simulink model "Nomto Model"  (R2022a)
settings: Solver=VariableStepAuto  StartTime=0.0  StopTime=200  RelTol=1e-3
settings Model: Creator=Z0150218  LastModifiedBy=Z0150218

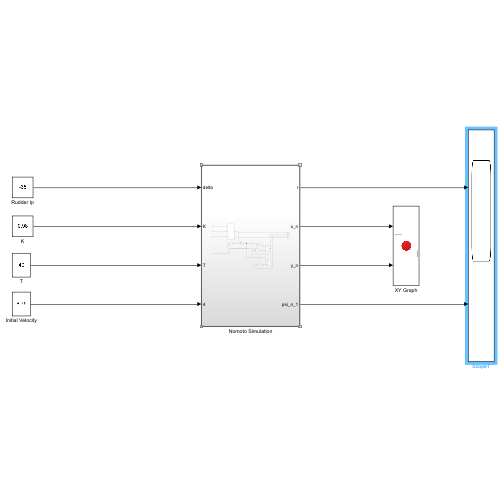
[thumbnail: Simulink's stored preview of the top-level diagram]
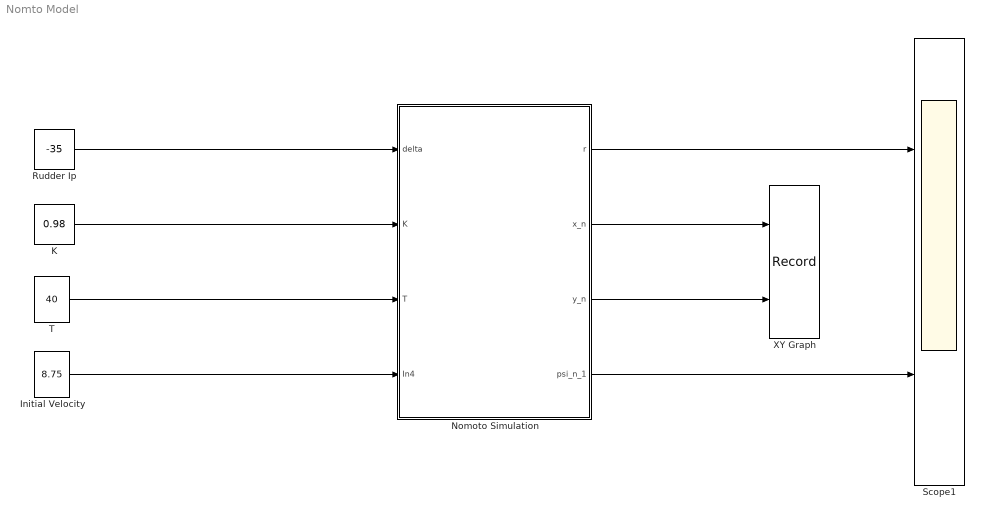
== system Nomto Model ==
  Initial Velocity : Constant  Value=8.75
  K : Constant  Value=0.98
  Nomoto Simulation : Subsystem
  Rudder Ip : Constant  Value=-35
  Scope1 : Scope  NumInputPorts=2
  T : Constant  Value=40
  XY Graph : Record  VariableName=X_Y_Position  RecordToWorkspace=on  FileSettingsInternal="{\"entries\":[{\"content\":{\"excelSettings\":{\"content\":{},\"type\":\"Streamout.ExcelSettings\"}},\"type\":\"Streamout.FileSettingStorage\",\"uuid\":\"6635f460-40b1-429d-8992-c5b395233bd7\"}],\"packageUris\":[\"http://schema.mathworks.com/mf0/streamout_blocks/R2020a\"],\"version\":\"1.0\"}"  Layout=[1 1]  SignalsInternal="{\"entries\":[{\"content\":{\"signals\":[{\"content\":{\"blockPath\":[\"model/XY Graph\"],\"channel\":[],\"dimensions\":[1],\"domain\":\"model/XY Graph\",\"lineColor\":\"#a2142f\",\"plots\":[1],\"port\":1,\"sid\":[\"\"],\"signalID\":43,\"signalName\":\"Nomoto Simulation:2\"},\"type\":\"RecordBlkView.Signal\",\"uuid\":\"2db5812d-c037-4b14-baed-b0e3edf6e0ba\"},{\"content\":{\"blockPath\":[\"model/XY Graph\"],\"channel\":[],\"dimensions\":[1],\"domain\":\"model/XY Graph\",\"lineColor\":\"#139fff\",\"plots\":[1],\"port\":2,\"sid\":[\"\"],\"signalID\":47,\"signalName\":\"Nomoto Simulation:3\"},\"type\":\"RecordBlkView.Signal\",\"uuid\":\"7fc5cd1a-1a78-4c0c-9b5d-9f5c7e47b2eb\"}]},\"type\":\"RecordBlkView.InputSignals\",\"uuid\":\"ea99f773-b7af-4dc6-9da2-234de1809b82\"}],\"packageUris\":[\"http://schema.mathworks.com/mf0/streamout_blocks/R2020a\"],\"version\":\"1.0\"}"  VisualizationBindings="{\"xyplotplugin\":{\"info\":[{\"series\":[{\"bindingParametersList\":[{\"parameter\":\"X-Axis\",\"signalID\":43,\"signalName\":\"Nomoto Simulation:2\"},{\"parameter\":\"Y-Axis\",\"signalID\":47,\"signalName\":\"Nomoto Simulation:3\"}],\"seriesID\":59298}],\"subplotID\":1}]}}"  CompatibilityTag=XY
  wires:
  Rudder Ip/1 -> Nomoto Simulation/1(delta)
  K/1 -> Nomoto Simulation/2(K)
  T/1 -> Nomoto Simulation/3(T)
  Initial Velocity/1 -> Nomoto Simulation/4(In4)
  Nomoto Simulation/4(psi_n_1) -> Scope1/2
  Nomoto Simulation/1(r) -> Scope1/1
  Nomoto Simulation/2(x_n) -> XY Graph/1
  Nomoto Simulation/3(y_n) -> XY Graph/2

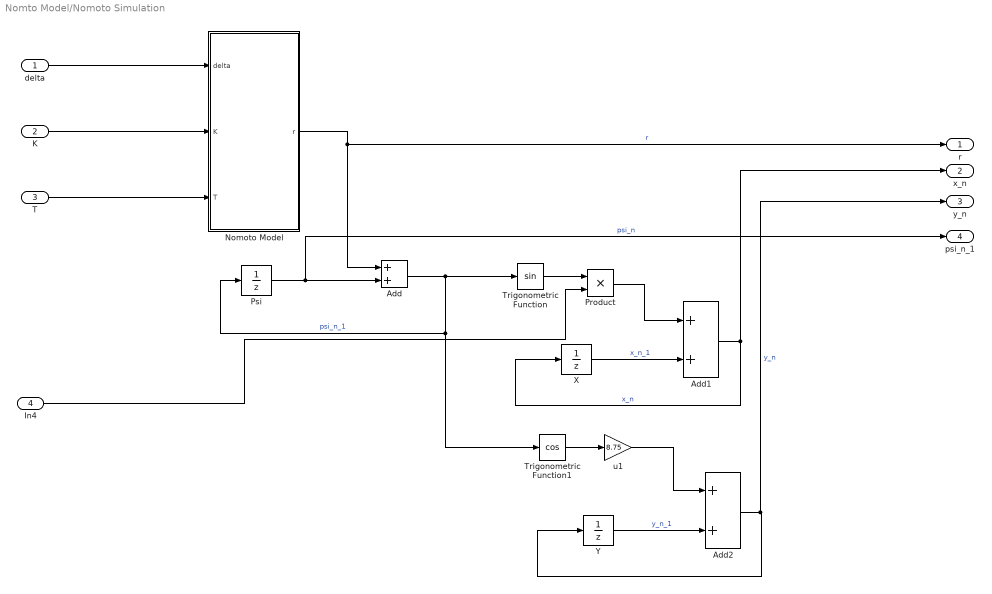
== system Nomto Model/Nomoto Simulation ==
  delta : Inport
  K : Inport  Port=2
  T : Inport  Port=3
  In4 : Inport  Port=4
  Add : Sum
  Add1 : Sum
  Add2 : Sum
  Nomoto Model : Subsystem
  Product : Product
  Psi : UnitDelay  SampleTime=-1  HasFrameUpgradeWarning=on
  Trigonometric Function : Trigonometry
  Trigonometric Function1 : Trigonometry  Operator=cos
  X : UnitDelay  SampleTime=-1  HasFrameUpgradeWarning=on
  Y : UnitDelay  SampleTime=-1  HasFrameUpgradeWarning=on
  u1 : Gain  Gain=8.75
  r : Outport
  x_n : Outport  Port=2
  y_n : Outport  Port=3
  psi_n_1 : Outport  Port=4
  wires:
  K/1 -> Nomoto Model/2(K)
  Add1/1 -> x_n/1, X/1  "x_n"
  Add/1 -> Trigonometric Function1/1, Psi/1, Trigonometric Function/1  "psi_n_1"
  Psi/1 -> psi_n_1/1, Add/2  "psi_n"
  Add2/1 -> y_n/1, Y/1  "y_n"
  Product/1 -> Add1/1
  Nomoto Model/1(r) -> r/1, Add/1  "r"
  In4/1 -> Product/2
  X/1 -> Add1/2  "x_n_1"
  Trigonometric Function/1 -> Product/1
  Trigonometric Function1/1 -> u1/1
  Y/1 -> Add2/2  "y_n_1"
  u1/1 -> Add2/1
  delta/1 -> Nomoto Model/1(delta)
  T/1 -> Nomoto Model/3(T)

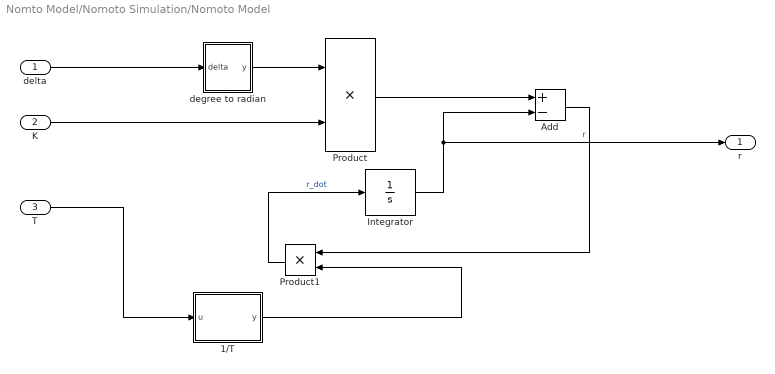
== system Nomto Model/Nomoto Simulation/Nomoto Model ==
  delta : Inport
  K : Inport  Port=2
  T : Inport  Port=3
  1/T : MATLAB Function  TreatAsAtomicUnit=on
  Add : Sum  Inputs=+-
  Integrator : Integrator
  Product : Product
  Product1 : Product
  degree to radian : MATLAB Function  TreatAsAtomicUnit=on
  r : Outport
  wires:
  T/1 -> 1/T/1(u)
  Integrator/1 -> r/1, Add/2  "r"
  delta/1 -> degree to radian/1(delta)
  1/T/1(y) -> Product1/2
  Add/1 -> Product1/1
  Product1/1 -> Integrator/1  "r_dot"
  degree to radian/1(y) -> Product/1
  K/1 -> Product/2
  Product/1 -> Add/1

== matlab function Nomto Model/Nomoto Simulation/Nomoto Model/degree to radian ==
  data: delta input; y output
function y = fcn(delta)

y = deg2rad(delta);

== matlab function Nomto Model/Nomoto Simulation/Nomoto Model/1//T ==
  data: u input; y output
function y = fcn(u)

y = 1/u;
